simulink model "IP02_CartOnTable"  (R2024b)
settings: Solver=ode45  StartTime=0.0  StopTime=10  MaxStep=1e-3  RelTol=1e-4  AbsTol=1e-6
undefined symbols (not defined in the file): A_input, f_input
settings Model: Creator=Karim Negm  LastModifiedBy=Karim Negm

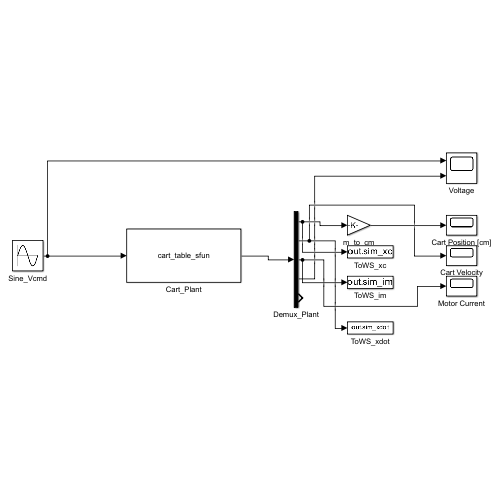
[thumbnail: Simulink's stored preview of the top-level diagram]
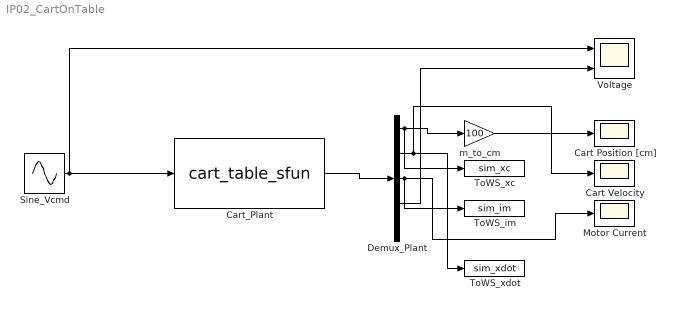
== system IP02_CartOnTable ==
  Cart Position [cm] : Scope
  Cart Velocity : Scope
  Cart_Plant : M-S-Function  FunctionName=cart_table_sfun
  Demux_Plant : Demux  Outputs=5
  Motor Current : Scope
  Sine_Vcmd : Sin  Amplitude=A_input  Frequency=2*pi*f_input  SampleTime=0
  ToWS_im : ToWorkspace  VariableName=sim_im  SaveFormat=Timeseries  SampleTime=-1
  ToWS_xc : ToWorkspace  VariableName=sim_xc  SaveFormat=Timeseries  SampleTime=-1
  ToWS_xdot : ToWorkspace  VariableName=sim_xdot  SaveFormat=Timeseries  SampleTime=-1
  Voltage : Scope  NumInputPorts=2
  m_to_cm : Gain  Gain=100
  wires:
  Sine_Vcmd/1 -> Cart_Plant/1, Voltage/1
  Cart_Plant/1 -> Demux_Plant/1
  Demux_Plant/1 -> m_to_cm/1, ToWS_xc/1
  m_to_cm/1 -> Cart Position [cm]/1
  Demux_Plant/2 -> Cart Velocity/1, ToWS_xdot/1
  Demux_Plant/3 -> Motor Current/1, ToWS_im/1
  Demux_Plant/4 -> Voltage/2
